simulink subsystem "PieroControladoPosicionZ"  (R2023b)
settings: Solver=VariableStepAuto  StartTime=0.0  StopTime=10.0  RelTol=1e-3
undefined symbols (not defined in the file): DiscIntNeverNeededParam
settings Model: Creator=Carlos  LastModifiedBy=Carlos

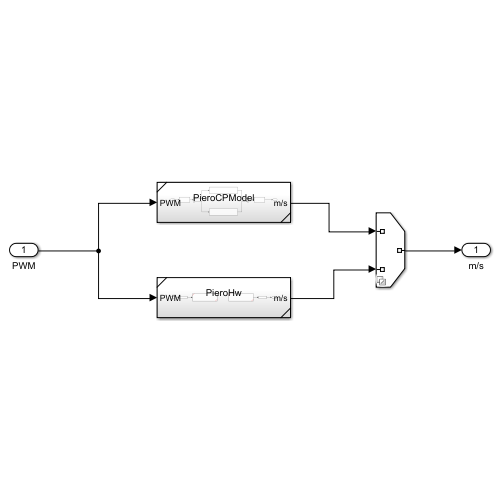
[thumbnail: Simulink's stored preview of the top-level diagram]
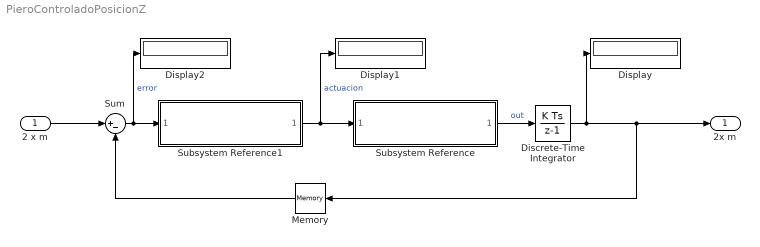
== system PieroControladoPosicionZ ==
  2 x m : Inport
  Discrete-Time Integrator : DiscreteIntegrator  SampleTime=-1  ICPrevOutput=DiscIntNeverNeededParam  ICPrevScaledInput=DiscIntNeverNeededParam
  Display : Display
  Display1 : Display
  Display2 : Display
  Memory : Memory
  Subsystem Reference : Subsystem  ReferencedSubsystem=PieroCPZ
  Subsystem Reference1 : Subsystem  ReferencedSubsystem=ControladorPosicion
  Sum : Sum  Inputs=|+-
  2x m : Outport
  wires:
  Subsystem Reference1/1 -> Subsystem Reference/1, Display1/1  "actuacion"
  2 x m/1 -> Sum/1
  Sum/1 -> Subsystem Reference1/1, Display2/1  "error"
  Subsystem Reference/1 -> Discrete-Time Integrator/1  "out"
  Memory/1 -> Sum/2
  Discrete-Time Integrator/1 -> 2x m/1, Memory/1, Display/1
